simulink library "modVehicle000_cl"  (R2018b)
settings: Solver=VariableStepAuto  StartTime=0.0  StopTime=10.0  RelTol=1e-3
undefined symbols (not defined in the file): constantVelBool, constantVelMag, MMAddBool, MMOverrideBool, simParam, vhcl
libraries: vrlib x1, eulAng2RotMat_ul x1, vectorNormalizer_ul x1, dragTurbine_ul x1, fluidDynamicSurface_cl x1, sixDoFDynamics_ul x1, tethersMoment_cl x1, thrAttachPtKinematics_ul x1
settings Model: Creator=mcobb  LastModifiedBy=jldanie5

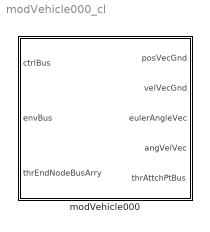
== system modVehicle000_cl ==
  modVehicle000 : Subsystem  VariantControl=VSS_vehicle_vehicle000  mask{vcl=vhcl, rho=simParam.env_param.density.Value, grav=simParam.env_param.grav.Value}
      mask prompts: vcl "Vehicle"; rho "Fuild Density"; grav "Gravity"
      mask DialogControl Container9 Prompt: General
      mask DialogControl Container5 Prompt: Vehicle object
      mask DialogControl ParameterGroupVar Prompt: Environmental
      mask Display:
      | image('kite.jpg',[100 100 601 528]/4,'on')
      | 
      | port_label('input',1,'ctrlBus')
      | port_label('input',2,'envBus')
      | port_label('input',3,'thrEndNodeBusArry')
      | 
      | port_label('output',1,'posVecGnd')
      | port_label('output',2,'velVecGnd')
      | port_label('output',3,'eulAng')
      | port_label('output',4,'angVelVec')
      | port_label('output',5,'thrAttchPtBus')

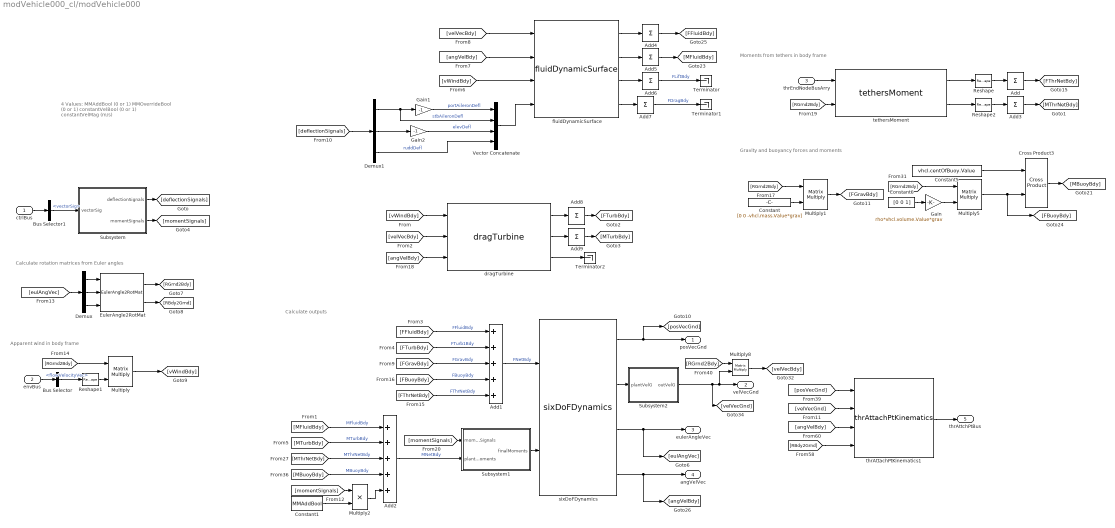
== system modVehicle000_cl/modVehicle000 ==
  note: 4 Values:
      | MMAddBool (0 or 1)
      | MMOverrideBool (0 or 1)
      | constantVelBool (0 or 1)
      | constantVelMag (m/s)
  note: Calculate outputs
  note: Apparent wind in body frame
  note: Calculate rotation matrices from Euler angles
  note: Gravity and buoyancy forces and moments
  note: Moments from tethers in body frame
  ctrlBus : Inport  OutDataTypeStr=Bus: ctrlBus
  envBus : Inport  Port=2  OutDataTypeStr=Bus: envBus
  thrEndNodeBusArry : Inport  Port=3
  Add : Sum  Inputs=+  CollapseMode=Specified dimension  CollapseDim=2
  Add1 : Sum  Inputs=+++++
  Add2 : Sum  Inputs=+++++
  Add3 : Sum  Inputs=+  CollapseMode=Specified dimension  CollapseDim=2
  Add{4..9} (6 alike) : Sum  Inputs=1  CollapseMode=Specified dimension  CollapseDim=2
  Bus Selector : BusSelector  OutputSignals=flowVelocityVec
  Bus Selector1 : BusSelector  OutputSignals=vectorSig
  Constant : Constant  Value=[0 0 -vhcl.mass.Value*grav]
  Constant1 : Constant  Value=MMAddBool
  Constant5 : Constant  Value=vhcl.centOfBuoy.Value
  Constant6 : Constant  Value=[0 0 1]
  Cross Product3 : vrlib/Utilities/Cross Product
      settings: SourceProductBaseCode=VR
  Demux : Demux  Outputs=3
  Demux1 : Demux  Outputs=3
  EulerAngle2RotMat : eulAng2RotMat_ul/EulerAngle2RotMat  SystemSampleTime=-1
  Gain : Gain  Gain=rho*vhcl.volume.Value*grav
  Gain1 : Gain  Gain=-1
  Gain2 : Gain  Gain=-1
  Multiply{,1,5,8} (4 alike) : Product  Multiplication=Matrix(*)
  Multiply2 : Product
  Reshape : Reshape  OutputDimensionality=Customize  OutputDimensions=[3 vhcl.numTethers.Value]
  Reshape1 : Reshape  OutputDimensionality=Column vector (2-D)
  Reshape2 : Reshape  OutputDimensionality=Customize  OutputDimensions=[3 vhcl.numTethers.Value]
  Subsystem : Subsystem
  Subsystem1 : Subsystem
  Subsystem2 : Subsystem
  Terminator : Terminator
  Terminator1 : Terminator
  Terminator2 : Terminator
  Vector Concatenate : Concatenate  NumInputs=4
  dragTurbine : dragTurbine_ul/dragTurbine  rho_fluid=rho  turb_struct=vhcl.struct('OCT.turb')
  fluidDynamicSurface : fluidDynamicSurface_cl/fluidDynamicSurface  aeroStruct=vcl.struct('OCT.aeroSurf')  fluidDensity=rho
  sixDoFDynamics : sixDoFDynamics_ul/sixDoFDynamics  M=vhcl.mass.Value  J=vhcl.inertia.Value  initPos=vhcl.initPosVecGnd.Value  initVel=vhcl.initVelVecGnd.Value  initEulAngs=vhcl.initEulAngBdy.Value  initAngVel=vhcl.initAngVelVecBdy.Value
  tethersMoment : tethersMoment_cl/tethersMoment  arms=vhcl.struct('OCT.thrAttch')
  thrAttachPtKinematics1 : thrAttachPtKinematics_ul/thrAttachPtKinematics  atchPts=vhcl.struct('OCT.thrAttch')
  posVecGnd : Outport
  velVecGnd : Outport  Port=2
  eulerAngleVec : Outport  Port=3
  angVelVec : Outport  Port=4
  thrAttchPtBus : Outport  Port=5
  wires:
  Bus Selector/1 -> Reshape1/1  "<flowVelocityVec>"
  [eulAngVec] -> Demux/1
  Demux/2 -> EulerAngle2RotMat/2
  Demux/1 -> EulerAngle2RotMat/1
  Demux/3 -> EulerAngle2RotMat/3
  EulerAngle2RotMat/1 -> [RGrnd2Bdy]
  EulerAngle2RotMat/2 -> [RBdy2Grnd]
  [RGrnd2Bdy] -> Multiply/1
  Multiply/1 -> [vWindBdy]
  [RGrnd2Bdy] -> Multiply1/1
  Multiply1/1 -> [FGravBdy]
  thrEndNodeBusArry/1 -> tethersMoment/1
  Constant6/1 -> Gain/1
  Multiply5/1 -> Cross Product3/2, [FBuoyBdy]
  [RGrnd2Bdy] -> Multiply5/1
  Cross Product3/1 -> [MBuoyBdy]
  Constant5/1 -> Cross Product3/1
  [MFluidBdy] -> Add2/1  "MFluidBdy"
  [MThrNetBdy] -> Add2/3  "MThrNetBdy"
  [MTurbBdy] -> Add2/2  "MTurbBdy"
  sixDoFDynamics/3 -> [eulAngVec], eulerAngleVec/1
  sixDoFDynamics/4 -> [angVelBdy], angVelVec/1
  [FFluidBdy] -> Add1/1  "FFluidBdy"
  [FTurbBdy] -> Add1/2  "FTurb1Bdy"
  Constant/1 -> Multiply1/2
  fluidDynamicSurface/2 -> Add5/1
  sixDoFDynamics/1 -> [posVecGnd], posVecGnd/1
  Multiply8/1 -> [velVecBdy]
  sixDoFDynamics/2 -> Subsystem2/1(plantVelG)
  [RGrnd2Bdy] -> Multiply8/1
  [angVelBdy] -> thrAttachPtKinematics1/3
  thrAttachPtKinematics1/1 -> thrAttchPtBus/1
  [posVecGnd] -> thrAttachPtKinematics1/1
  [RBdy2Grnd] -> thrAttachPtKinematics1/4
  [velVecGnd] -> thrAttachPtKinematics1/2
  tethersMoment/1 -> Reshape/1
  Reshape/1 -> Add/1
  Add/1 -> [FThrNetBdy]
  [RGrnd2Bdy] -> tethersMoment/2
  Reshape1/1 -> Multiply/2
  Add3/1 -> [MThrNetBdy]
  Reshape2/1 -> Add3/1
  tethersMoment/2 -> Reshape2/1
  Add1/1 -> sixDoFDynamics/1  "FNetBdy"
  envBus/1 -> Bus Selector/1
  fluidDynamicSurface/1 -> Add4/1
  fluidDynamicSurface/3 -> Add6/1
  fluidDynamicSurface/4 -> Add7/1
  [vWindBdy] -> fluidDynamicSurface/3
  [angVelBdy] -> fluidDynamicSurface/2
  [velVecBdy] -> fluidDynamicSurface/1
  Add4/1 -> [FFluidBdy]
  Add5/1 -> [MFluidBdy]
  Add6/1 -> Terminator/1  "FLiftBdy"
  Add7/1 -> Terminator1/1  "FDragBdy"
  dragTurbine/1 -> Add8/1
  dragTurbine/2 -> Add9/1
  Add8/1 -> [FTurbBdy]
  Add9/1 -> [MTurbBdy]
  dragTurbine/3 -> Terminator2/1
  [vWindBdy] -> dragTurbine/1
  [velVecBdy] -> dragTurbine/2
  [angVelBdy] -> dragTurbine/3
  [MBuoyBdy] -> Add2/4  "MBuoyBdy"
  [FThrNetBdy] -> Add1/5  "FThrNetBdy"
  [FBuoyBdy] -> Add1/4  "FBuoyBdy"
  [FGravBdy] -> Add1/3  "FGravBdy"
  Gain/1 -> Multiply5/2
  Vector Concatenate/1 -> fluidDynamicSurface/4
  ctrlBus/1 -> Bus Selector1/1
  [deflectionSignals] -> Demux1/1
  Demux1/3 -> Vector Concatenate/4  "ruddDefl"
  Demux1/2 -> Gain2/1
  Gain1/1 -> Vector Concatenate/1  "portAileronDefl"
  Demux1/1 -> Vector Concatenate/2, Gain1/1  "stbAileronDefl"
  Gain2/1 -> Vector Concatenate/3  "elevDefl"
  Bus Selector1/1 -> Subsystem/1(vectorSig)  "<vectorSig>"
  Subsystem/1(deflectionSignals) -> [deflectionSignals]
  Subsystem/2(momentSignals) -> [momentSignals]
  Subsystem1/1(finalMoments) -> sixDoFDynamics/2
  Add2/1 -> Subsystem1/2(plantCreatedMoments)  "MNetBdy"
  [momentSignals] -> Subsystem1/1(momentSignals)
  Subsystem2/1(outVelG) -> velVecGnd/1, Multiply8/2, [velVecGnd]
  [momentSignals] -> Multiply2/1
  Multiply2/1 -> Add2/5
  Constant1/1 -> Multiply2/2

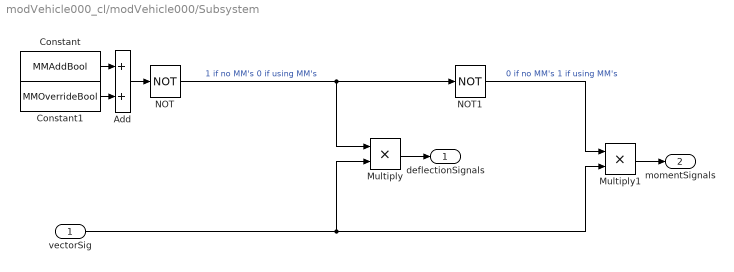
== system modVehicle000_cl/modVehicle000/Subsystem ==
  vectorSig : Inport
  Add : Sum
  Constant : Constant  Value=MMAddBool
  Constant1 : Constant  Value=MMOverrideBool
  Multiply : Product
  Multiply1 : Product
  NOT : Logic  Operator=NOT  IconShape=distinctive  AllPortsSameDT=off  OutDataTypeStr=boolean
  NOT1 : Logic  Operator=NOT  IconShape=distinctive  AllPortsSameDT=off  OutDataTypeStr=boolean
  deflectionSignals : Outport
  momentSignals : Outport  Port=2
  wires:
  Multiply/1 -> deflectionSignals/1
  Constant/1 -> Add/1
  Constant1/1 -> Add/2
  Add/1 -> NOT/1
  NOT/1 -> NOT1/1, Multiply/1  "1 if no MM's 0 if using MM's"
  Multiply1/1 -> momentSignals/1
  NOT1/1 -> Multiply1/1  "0 if no MM's 1 if using MM's"
  vectorSig/1 -> Multiply1/2, Multiply/2

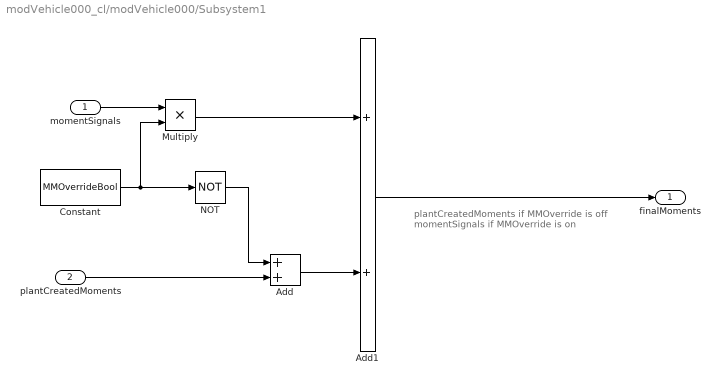
== system modVehicle000_cl/modVehicle000/Subsystem1 ==
  note: plantCreatedMoments if MMOverride is off
      | momentSignals if MMOverride is on
  momentSignals : Inport
  plantCreatedMoments : Inport  Port=2
  Add : Sum
  Add1 : Sum
  Constant : Constant  Value=MMOverrideBool
  Multiply : Product
  NOT : Logic  Operator=NOT  IconShape=distinctive  AllPortsSameDT=off  OutDataTypeStr=boolean
  finalMoments : Outport
  wires:
  Constant/1 -> Multiply/2, NOT/1
  momentSignals/1 -> Multiply/1
  plantCreatedMoments/1 -> Add/2
  NOT/1 -> Add/1
  Add/1 -> Add1/2
  Multiply/1 -> Add1/1
  Add1/1 -> finalMoments/1

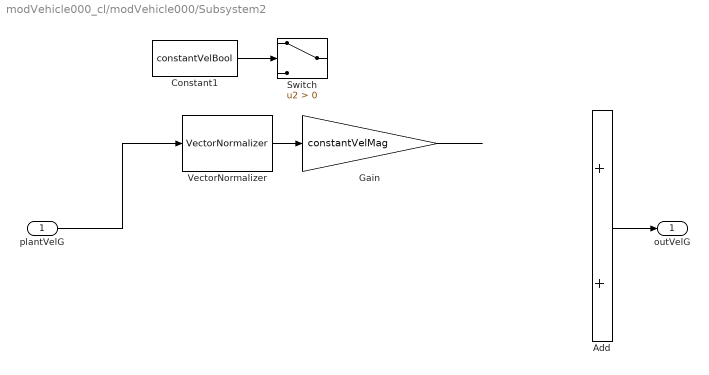
== system modVehicle000_cl/modVehicle000/Subsystem2 ==
  plantVelG : Inport
  Add : Sum
  Constant1 : Constant  Value=constantVelBool
  Gain : Gain  Gain=constantVelMag
  Switch : Switch  Criteria=u2 > Threshold
  "VectorNormalizer " : vectorNormalizer_ul/VectorNormalizer   SystemSampleTime=-1
  outVelG : Outport
  wires:
  plantVelG/1 -> "VectorNormalizer "/1
  "VectorNormalizer "/1 -> Gain/1
  Gain/1 -> ?
  ? -> Add/1
  Add/1 -> outVelG/1
  Constant1/1 -> Switch/2
